simulink model "BibelPunktMasse"  (R2022a)
settings: Solver=VariableStepAuto  StartTime=0.0  StopTime=simtime  RelTol=1e-3
values from neighbouring files (symbols this model uses):
  AVeh = 1.05    [first_test.mat]    (also in malgucka.m)
  coeffAir = 1.35    [first_test.mat]    (also in malgucka.m)
  coeffLift = 5.2    [first_test.mat]    (also in malgucka.m)
  densAir = 1.225    [first_test.mat]    (also in malgucka.m)
  dstRdTir = 0.2032    [first_test.mat]    (also in malgucka.m)
  gbx = 16    [first_test.mat]    (also in malgucka.m = 13.11)
  IMot = 1    [first_test.mat]    (also in malgucka.m = 2)
  initial_speed = max(v_acc) / 3.6    [laptimeV1.m]
  initial_whlspeed = 0    [laptimeV1.m]
  IWhl = 2    [first_test.mat]    (also in malgucka.m = 3)
  mVeh = 282    [first_test.mat]    (also in malgucka.m)
  tq_Mot_Re = [40 40 40 40 40 40 40 40 40 40 40 40 ... (46 elements, 1x46)]    [first_test.mat]    (also in laptimeV1.m = [0 0 0 0 0 0 0])
libraries: mfeval_LIB x4
settings Model: Creator=gbour  LastModifiedBy=gbour

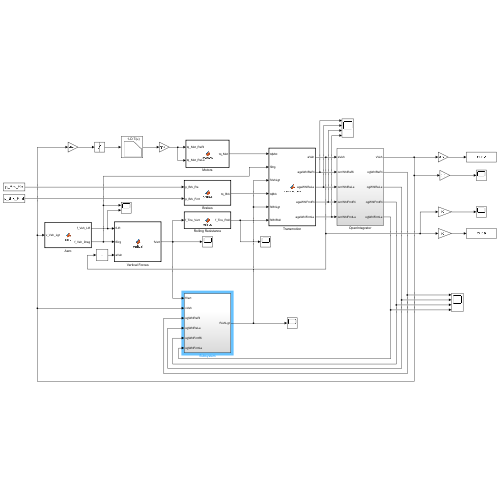
[thumbnail: Simulink's stored preview of the top-level diagram]
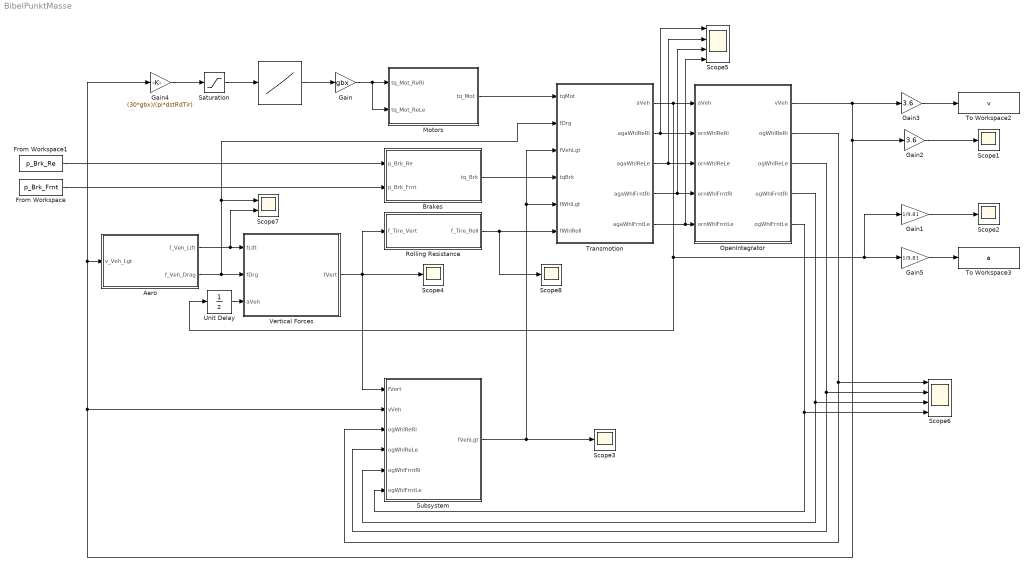
== system BibelPunktMasse ==
  " " : Lookup_n-D  NumberOfTableDimensions=1  BreakpointsForDimension1=[0 100 12000 15000 20000 22500 22501]  Table=tq_Mot_Re  InternalRulePriority=Speed  RndMeth=Simplest
  Aero : MATLAB Function  TreatAsAtomicUnit=on
  Brakes : MATLAB Function  TreatAsAtomicUnit=on
  From Workspace : FromWorkspace  VariableName=p_Brk_Frnt
  From Workspace1 : FromWorkspace  VariableName=p_Brk_Re
  Gain : Gain  Gain=gbx
  Gain1 : Gain  Gain=1/9.81
  Gain2 : Gain  Gain=3.6
  Gain3 : Gain  Gain=3.6
  Gain4 : Gain  Gain=(30*gbx)/(pi*dstRdTir)
  Gain5 : Gain  Gain=1/9.81
  Motors : MATLAB Function  TreatAsAtomicUnit=on
  OpenIntegrator : Subsystem
  Rolling Resistance : MATLAB Function  TreatAsAtomicUnit=on
  Saturation : Saturate  UpperLimit=22501  LowerLimit=0
  Scope{1..4,8} (5 alike) : Scope
  Scope5 : Scope  NumInputPorts=4
  Scope6 : Scope  NumInputPorts=4
  Scope7 : Scope  NumInputPorts=2
  Subsystem : Subsystem
  To Workspace2 : ToWorkspace  VariableName=v  SampleTime=-1
      settings: Save2DSignal=2-D array (concatenate along first dimension)
  To Workspace3 : ToWorkspace  VariableName=a  SampleTime=-1
      settings: Save2DSignal=2-D array (concatenate along first dimension)
  Transmotion : MATLAB Function  TreatAsAtomicUnit=on
  Unit Delay : UnitDelay  SampleTime=-1  HasFrameUpgradeWarning=on
  Vertical Forces : MATLAB Function  TreatAsAtomicUnit=on
  wires:
  OpenIntegrator/1(vVeh) -> Gain3/1, Subsystem/2(vVeh), Gain4/1, Aero/1(v_Veh_Lgt), Gain2/1
  Transmotion/5(agaWhlFrntLe) -> Scope5/4, OpenIntegrator/5(ornWhlFrntLe)
  Transmotion/1(aVeh) -> Gain1/1, Gain5/1, Unit Delay/1, OpenIntegrator/1(aVeh)
  Transmotion/2(agaWhlReRi) -> OpenIntegrator/2(ornWhlReRi), Scope5/1
  Transmotion/3(agaWhlReLe) -> OpenIntegrator/3(ornWhlReLe), Scope5/2
  Transmotion/4(agaWhlFrntRi) -> OpenIntegrator/4(ornWhlFrntRi), Scope5/3
  Brakes/1(tq_Brk) -> Transmotion/4(tqBrk)
  From Workspace1/1 -> Brakes/1(p_Brk_Re)
  From Workspace/1 -> Brakes/2(p_Brk_Frnt)
  Rolling Resistance/1(f_Tire_Roll) -> Scope8/1, Transmotion/6(fWhlRoll)
  Aero/2(f_Veh_Drag) -> Vertical Forces/2(fDrg), Transmotion/2(fDrg), Scope7/1
  Vertical Forces/1(fVert) -> Subsystem/1(fVert), Scope4/1, Rolling Resistance/1(f_Tire_Vert)
  Aero/1(f_Veh_Lift) -> Scope7/2, Vertical Forces/1(fLift)
  Unit Delay/1 -> Vertical Forces/3(aVeh)
  Subsystem/1(fVehLgt) -> Transmotion/5(fWhlLgt), Transmotion/3(fVehLgt), Scope3/1
  OpenIntegrator/2(ogWhlReRi) -> Subsystem/3(ogWhlReRi), Scope6/1
  OpenIntegrator/3(ogWhlReLe) -> Subsystem/4(ogWhlReLe), Scope6/2
  OpenIntegrator/4(ogWhlFrntRi) -> Subsystem/5(ogWhlFrntRi), Scope6/3
  OpenIntegrator/5(ogWhlFrntLe) -> Subsystem/6(ogWhlFrntLe), Scope6/4
  Motors/1(tq_Mot) -> Transmotion/1(tqMot)
  Saturation/1 -> " "/1
  Gain4/1 -> Saturation/1
  Gain/1 -> Motors/2(tq_Mot_ReLe), Motors/1(tq_Mot_ReRi)
  " "/1 -> Gain/1
  Gain2/1 -> Scope1/1
  Gain3/1 -> To Workspace2/1
  Gain5/1 -> To Workspace3/1
  Gain1/1 -> Scope2/1

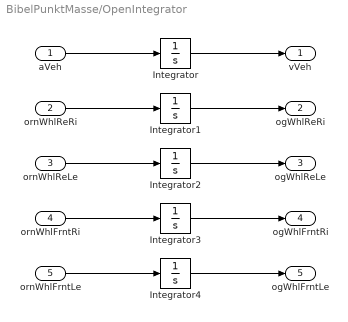
== system BibelPunktMasse/OpenIntegrator ==
  aVeh : Inport
  ornWhlReRi : Inport  Port=2
  ornWhlReLe : Inport  Port=3
  ornWhlFrntRi : Inport  Port=4
  ornWhlFrntLe : Inport  Port=5
  Integrator : Integrator  InitialCondition=initial_speed
  Integrator{1..4} (4 alike) : Integrator  InitialCondition=initial_whlspeed
  vVeh : Outport
  ogWhlReRi : Outport  Port=2
  ogWhlReLe : Outport  Port=3
  ogWhlFrntRi : Outport  Port=4
  ogWhlFrntLe : Outport  Port=5
  wires:
  aVeh/1 -> Integrator/1
  Integrator/1 -> vVeh/1
  ornWhlReRi/1 -> Integrator1/1
  ornWhlReLe/1 -> Integrator2/1
  ornWhlFrntRi/1 -> Integrator3/1
  ornWhlFrntLe/1 -> Integrator4/1
  Integrator1/1 -> ogWhlReRi/1
  Integrator2/1 -> ogWhlReLe/1
  Integrator3/1 -> ogWhlFrntRi/1
  Integrator4/1 -> ogWhlFrntLe/1

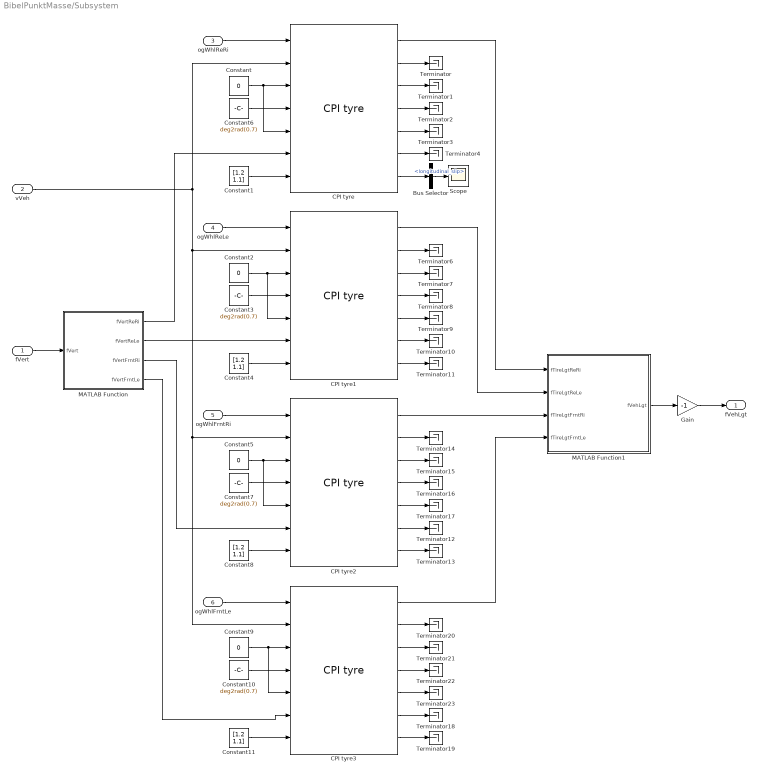
== system BibelPunktMasse/Subsystem ==
  fVert : Inport
  vVeh : Inport  Port=2
  ogWhlReRi : Inport  Port=3
  ogWhlReLe : Inport  Port=4
  ogWhlFrntRi : Inport  Port=5
  ogWhlFrntLe : Inport  Port=6
  Bus Selector : BusSelector  OutputSignals=longitudinal_slip
  CPI tyre : mfeval_LIB/CPI tyre  Description=Magic Formula 6.1.2 tyre model including relaxation length and transient calculations  userParameterSource='model.tir'  userSide=2 right  userDynamics=1 steady state  userUseMode=1 combined  enablePressure=on  userPressure=0.82
      settings: SourceProductName=MFeval Library
  CPI tyre1 : mfeval_LIB/CPI tyre  Description=Magic Formula 6.1.2 tyre model including relaxation length and transient calculations  userParameterSource='model.tir'  userSide=1 left  userDynamics=1 steady state  userUseMode=1 combined  enablePressure=on  userPressure=0.82
      settings: SourceProductName=MFeval Library
  CPI tyre2 : mfeval_LIB/CPI tyre  Description=Magic Formula 6.1.2 tyre model including relaxation length and transient calculations  userParameterSource='model.tir'  userSide=2 right  userDynamics=1 steady state  userUseMode=1 combined  enablePressure=on  userPressure=0.82
      settings: SourceProductName=MFeval Library
  CPI tyre3 : mfeval_LIB/CPI tyre  Description=Magic Formula 6.1.2 tyre model including relaxation length and transient calculations  userParameterSource='model.tir'  userSide=1 left  userDynamics=1 steady state  userUseMode=1 combined  enablePressure=on  userPressure=0.82
      settings: SourceProductName=MFeval Library
  Constant{,2,5,9} (4 alike) : Constant  Value=0
  Constant{1,4,8,11} (4 alike) : Constant  Value=[1.2 1.1]
  Constant{3,6..7,10} (4 alike) : Constant  Value=deg2rad(0.7)
  Gain : Gain  Gain=-1
  MATLAB Function : MATLAB Function  TreatAsAtomicUnit=on
  MATLAB Function1 : MATLAB Function  TreatAsAtomicUnit=on
  Scope : Scope
  Terminator{,1..4,6..23} (23 alike) : Terminator
  fVehLgt : Outport
  wires:
  ogWhlReRi/1 -> CPI tyre/1
  vVeh/1 -> CPI tyre/2, CPI tyre2/2, CPI tyre3/2, CPI tyre1/2
  Constant/1 -> CPI tyre/5, CPI tyre/3
  MATLAB Function/1(fVertReRi) -> CPI tyre/6
  Constant1/1 -> CPI tyre/7
  ogWhlReLe/1 -> CPI tyre1/1
  Constant2/1 -> CPI tyre1/5, CPI tyre1/3
  Constant3/1 -> CPI tyre1/4
  MATLAB Function/2(fVertReLe) -> CPI tyre1/6
  Constant4/1 -> CPI tyre1/7
  ogWhlFrntRi/1 -> CPI tyre2/1
  Constant5/1 -> CPI tyre2/5, CPI tyre2/3
  Constant6/1 -> CPI tyre/4
  Constant7/1 -> CPI tyre2/4
  MATLAB Function/3(fVertFrntRi) -> CPI tyre2/6
  Constant8/1 -> CPI tyre2/7
  ogWhlFrntLe/1 -> CPI tyre3/1
  Constant9/1 -> CPI tyre3/5, CPI tyre3/3
  Constant10/1 -> CPI tyre3/4
  Constant11/1 -> CPI tyre3/7
  MATLAB Function/4(fVertFrntLe) -> CPI tyre3/6
  CPI tyre/2 -> Terminator/1
  CPI tyre/3 -> Terminator1/1
  CPI tyre/4 -> Terminator2/1
  CPI tyre/5 -> Terminator3/1
  CPI tyre/6 -> Terminator4/1
  CPI tyre/7 -> Bus Selector/1
  CPI tyre1/7 -> Terminator11/1
  CPI tyre1/6 -> Terminator10/1
  CPI tyre1/5 -> Terminator9/1
  CPI tyre1/4 -> Terminator8/1
  CPI tyre1/3 -> Terminator7/1
  CPI tyre1/2 -> Terminator6/1
  CPI tyre2/7 -> Terminator13/1
  CPI tyre2/6 -> Terminator12/1
  CPI tyre2/5 -> Terminator17/1
  CPI tyre2/4 -> Terminator16/1
  CPI tyre2/3 -> Terminator15/1
  CPI tyre2/2 -> Terminator14/1
  CPI tyre3/2 -> Terminator20/1
  CPI tyre3/3 -> Terminator21/1
  CPI tyre3/4 -> Terminator22/1
  CPI tyre3/5 -> Terminator23/1
  CPI tyre3/6 -> Terminator18/1
  CPI tyre3/7 -> Terminator19/1
  CPI tyre/1 -> MATLAB Function1/1(fTireLgtReRi)
  CPI tyre1/1 -> MATLAB Function1/2(fTireLgtReLe)
  CPI tyre2/1 -> MATLAB Function1/3(fTireLgtFrntRi)
  CPI tyre3/1 -> MATLAB Function1/4(fTireLgtFrntLe)
  MATLAB Function1/1(fVehLgt) -> Gain/1
  fVert/1 -> MATLAB Function/1(fVert)
  Gain/1 -> fVehLgt/1
  Bus Selector/1 -> Scope/1  "<longitudinal_slip>"

== matlab function BibelPunktMasse/Motors ==
  data: tq_Mot_ReRi input size=1; tq_Mot output size=[4 1]; tq_Mot_ReLe input size=1
function tq_Mot = motors(tq_Mot_ReRi, tq_Mot_ReLe)

tq_Mot = zeros(4, 1);

tq_Mot(1) = tq_Mot_ReRi;
tq_Mot(2) = tq_Mot_ReLe;

end

== matlab function BibelPunktMasse/Vertical Forces ==
  data: fLift input size=1; fVert output size=[4 1]; fDrg input size=1; aVeh input size=1; mVeh parameter size=1
function fVert = vertical(fLift, fDrg, aVeh, mVeh)

fVert = zeros([4 1]);

fVert(1) = 0.26 * fLift + 0.05 * fDrg + 0.53/2 * 9.81 * mVeh + aVeh * 0.53/1.535 * mVeh * 0.5;

fVert(2) = 0.26 * fLift + 0.05 * fDrg + 0.53/2 * 9.81 * mVeh + aVeh * 0.53/1.535 * mVeh * 0.5;

fVert(3) = 0.24 * fLift - 0.05 * fDrg + 0.47/2 * 9.81 * mVeh - aVeh * 0.47/1.535 * mVeh * 0.5;

fVert(4) = 0.24 * fLift - 0.05 * fDrg + 0.47/2 * 9.81 * mVeh - aVeh * 0.47/1.535 * mVeh * 0.5;

end

== matlab function BibelPunktMasse/Transmotion ==
  data: tqMot input size=[4 1]; fDrg input size=1; fVehLgt input size=[4 1]; aVeh output size=1; agaWhlReRi output size=1; agaWhlReLe output size=1; agaWhlFrntRi output size=1; agaWhlFrntLe output size=1; tqBrk input size=[4 1]; fWhlLgt input size=[4 1]; fWhlRoll input size=[4 1]; mVeh parameter size=1; dstRdTir parameter size=1; IWhl parameter; IMot parameter; gbx parameter
function [aVeh, agaWhlReRi, agaWhlReLe, agaWhlFrntRi, agaWhlFrntLe] = transmotion(tqMot, fDrg, fVehLgt, tqBrk, fWhlLgt, fWhlRoll, mVeh, dstRdTir, IWhl, IMot, gbx)

aVeh = (1 / mVeh) * sum(fVehLgt - fDrg);

agaWhlReRi = (gbx * tqMot(1) + tqBrk(1) - (fWhlRoll(1) - fWhlLgt(1)) * dstRdTir) / (IWhl + gbx^2 * IMot);

agaWhlReLe = (gbx * tqMot(2) + tqBrk(2) - (fWhlRoll(2) - fWhlLgt(2)) * dstRdTir) / (IWhl + gbx^2 * IMot);

agaWhlFrntRi = (tqBrk(3) - (fWhlRoll(3) - fWhlLgt(3)) * dstRdTir) / (IWhl);

agaWhlFrntLe = (tqBrk(4) - (fWhlRoll(4) - fWhlLgt(4)) * dstRdTir) / (IWhl);

end

== matlab function BibelPunktMasse/Aero ==
  data: v_Veh_Lgt input size=1; f_Veh_Lift output size=1; f_Veh_Drag output size=1; densAir parameter size=1; AVeh parameter size=1; coeffLift parameter size=1; coeffAir parameter size=1
function [f_Veh_Lift, f_Veh_Drag] = aero(v_Veh_Lgt, densAir, AVeh, coeffLift, coeffAir)

f_Veh_Lift = 0.5 * densAir * AVeh * coeffLift * v_Veh_Lgt^2;
f_Veh_Drag = 0.5 * densAir * AVeh * coeffAir * v_Veh_Lgt^2;

end

== matlab function BibelPunktMasse/Subsystem/MATLAB Function ==
  data: fVert input size=[4 1]; fVertReRi output size=1; fVertReLe output size=1; fVertFrntRi output size=1; fVertFrntLe output size=1
function [fVertReRi, fVertReLe, fVertFrntRi, fVertFrntLe] = fcn(fVert)

fVertReRi = fVert(1);
fVertReLe = fVert(2);
fVertFrntRi = fVert(3);
fVertFrntLe = fVert(4);

end

== matlab function BibelPunktMasse/Subsystem/MATLAB Function1 ==
  data: fTireLgtReRi input size=1; fVehLgt output size=[4 1]; fTireLgtReLe input size=1; fTireLgtFrntRi input size=1; fTireLgtFrntLe input size=1
function fVehLgt = fcn(fTireLgtReRi, fTireLgtReLe, fTireLgtFrntRi, fTireLgtFrntLe)

fVehLgt = zeros([4 1]);

fVehLgt(1) = fTireLgtReRi;
fVehLgt(2) = fTireLgtReLe;
fVehLgt(3) = fTireLgtFrntRi;
fVehLgt(4) = fTireLgtFrntLe;

== matlab function BibelPunktMasse/Rolling Resistance ==
  data: f_Tire_Vert input size=[4 1]; f_Tire_Roll output size=[4 1]; coeffRoll parameter size=1
function f_Tire_Roll = rollres(f_Tire_Vert, coeffRoll)

f_Tire_Roll = f_Tire_Vert * coeffRoll;

end

== matlab function BibelPunktMasse/Brakes ==
  data: p_Brk_Re input size=1; tq_Brk output size=[4 1]; p_Brk_Frnt input size=1
function tq_Brk = brakes(p_Brk_Re, p_Brk_Frnt)

diam_Pist_Re = 25.4;        % piston diameter rear [mm]
nu_Pist_Re = 4;             % number of pistons rear
rad_BrkDisc_Re = 0.1725;    % brakedisc radius rear [m]
diam_Pist_Frnt = 25.4;      % piston diameter rear [mm]
nu_Pist_Frnt = 4;           % number of pistons rear
rad_BrkDisc_Frnt = 0.1725;  % brakedisc radius rear [m]
mu_Brk = 0.56;              % brake friction coefficient

tq_Brk = zeros(4, 1);

tq_Brk(1) = - 0.5 * (((pi * p_Brk_Re * ((diam_Pist_Re^2) / 4)) * nu_Pist_Re * mu_Brk) * 0.5 * rad_BrkDisc_Re);
tq_Brk(2) = - 0.5 * (((pi * p_Brk_Re * ((diam_Pist_Re^2) / 4)) * nu_Pist_Re * mu_Brk) * 0.5 * rad_BrkDisc_Re);
tq_Brk(3) = - 0.5 * (((pi * p_Brk_Frnt * ((diam_Pist_Frnt^2) / 4)) * nu_Pist_Frnt * mu_Brk) * 0.5 * rad_BrkDisc_Frnt);
tq_Brk(4) = - 0.5 * (((pi * p_Brk_Frnt * ((diam_Pist_Frnt^2) / 4)) * nu_Pist_Frnt * mu_Brk) * 0.5 * rad_BrkDisc_Frnt);

end
